simulink model "uavWaypointFollowing_HIL"  (R2021a)
settings: Solver=FixedStepDiscrete  StartTime=0.0  StopTime=10.0  RelTol=1e-3
values from neighbouring files (symbols this model uses):
  DEG2RAD = 0.0174533    [uavWaypointFollowing_HIL_Init_control.m]
  Kd_PITCH_AngleRate = 0.001    [uavWaypointFollowing_HIL_Init_control.m]
  Kd_ROLL_AngleRate = 0.001    [uavWaypointFollowing_HIL_Init_control.m]
  Kd_YAW_AngleRate = 0.00    (= 0)    [uavWaypointFollowing_HIL_Init_control.m]
  Ki_PITCH_AngleRate = 0.02    [uavWaypointFollowing_HIL_Init_control.m]
  Ki_ROLL_AngleRate = 0.02    [uavWaypointFollowing_HIL_Init_control.m]
  Ki_YAW_AngleRate = 0.001    [uavWaypointFollowing_HIL_Init_control.m]
  Kp_PITCH_ANGLE = 6.5    [uavWaypointFollowing_HIL_Init_control.m]
  Kp_PITCH_AngleRate = 0.1    [uavWaypointFollowing_HIL_Init_control.m]
  Kp_ROLL_ANGLE = 6.5    [uavWaypointFollowing_HIL_Init_control.m]
  Kp_ROLL_AngleRate = 0.1    [uavWaypointFollowing_HIL_Init_control.m]
  Kp_YAW_AngleRate = 0.3    [uavWaypointFollowing_HIL_Init_control.m]
  Kpxp = 1.0    (= 1)    [uavWaypointFollowing_HIL_Init_control.m]
  Kpyp = 1.0    (= 1)    [uavWaypointFollowing_HIL_Init_control.m]
  Kpzp = 4.0    (= 4)    [uavWaypointFollowing_HIL_Init_control.m]
  Kvxd = 0.01    [uavWaypointFollowing_HIL_Init_control.m]
  Kvxi = 0.4    [uavWaypointFollowing_HIL_Init_control.m]
  Kvxp = 2.5    [uavWaypointFollowing_HIL_Init_control.m]
  Kvyd = 0.01    [uavWaypointFollowing_HIL_Init_control.m]
  Kvyi = 0.4    [uavWaypointFollowing_HIL_Init_control.m]
  Kvyp = 2.5    [uavWaypointFollowing_HIL_Init_control.m]
  Kvzd = 0.005    [uavWaypointFollowing_HIL_Init_control.m]
  Kvzi = 0.01    [uavWaypointFollowing_HIL_Init_control.m]
  Kvzp = 0.45    [uavWaypointFollowing_HIL_Init_control.m]
  MAX_CONTROL_ANGLE_PITCH = 35    [uavWaypointFollowing_HIL_Init_control.m]
  MAX_CONTROL_ANGLE_RATE_PITCH = 220    [uavWaypointFollowing_HIL_Init_control.m]
  MAX_CONTROL_ANGLE_RATE_ROLL = 220    [uavWaypointFollowing_HIL_Init_control.m]
  MAX_CONTROL_ANGLE_RATE_Y = 200    [uavWaypointFollowing_HIL_Init_control.m]
  MAX_CONTROL_ANGLE_ROLL = 35    [uavWaypointFollowing_HIL_Init_control.m]
  MAX_CONTROL_VELOCITY_XY = 5    [uavWaypointFollowing_HIL_Init_control.m]
  MAX_CONTROL_VELOCITY_Z = 3    [uavWaypointFollowing_HIL_Init_control.m]
  Saturation_I_ah = 3.43    [uavWaypointFollowing_HIL_Init_control.m]
  Saturation_I_az = 5    [uavWaypointFollowing_HIL_Init_control.m]
  Saturation_I_RP_Max = 0.3    [uavWaypointFollowing_HIL_Init_control.m]
  Saturation_I_RP_Min = -0.3    [uavWaypointFollowing_HIL_Init_control.m]
  Saturation_I_Y_Max = 0.2    [uavWaypointFollowing_HIL_Init_control.m]
  Saturation_I_Y_Min = -0.2    [uavWaypointFollowing_HIL_Init_control.m]
  THR_HOVER = 0.609    [uavWaypointFollowing_HIL_Init_control.m]
undefined symbols (not defined in the file or in its folder): DiscIntNeverNeededParam, RGBLED_COLOR_ENUM, RGBLED_MODE_ENUM
libraries: simulink x7, pixhawk_slib_sensors_actuators x4, pixhawk_slib_uORB_RW x2
(part 2 of 2)

== matlab function uavWaypointFollowing_HIL/Control System/Subsystem/position_control/MATLAB Function ==
  data: eax input; eay input; psi input; phi output; theta output
function [phi, theta] = fcn(eax, eay, psi)
%Function description:
%  Convert the desired horizontal acceleration to the desired attitude angle
%Input:
%  eax, eaxy: desired horizontal acceleration
%  psi: yaw
%Output:
%  phi, theta: desired roll angle and desired pitch angle
g = 9.8;
phi = (-sin(psi)*eax + cos(psi)*eay)/g;
theta = (-cos(psi)*eax - sin(psi)*eay)/g;

== matlab function uavWaypointFollowing_HIL/Control System/InputConditioning1/deadzone4 ==
  data: u input; y output
function y = fcn(u)
%Function description:
%  Control the range of the remote control input from RCMin to RCMax, and
%  set a dead zone with a dead zone size of ±deadZone. The output y is
%  normalized to 0~1.You can get the RC calibration parameters in QGC.
RCMin = 1100;
RCMax = 1900;
RCMid = (RCMin + RCMax)/2;
deadZoneRate = 0.05;
deadZone = deadZoneRate*(RCMax - RCMin);
k = 1/(RCMax - RCMid - deadZone);
% saturation
if(u < RCMin)
    u = RCMin;
elseif(u > RCMax)
    u = RCMax;
end
% dead zone and normalize
 if(u > RCMid + deadZone)
    y = (u-RCMid - deadZone)*k;
 elseif(u < RCMid - deadZone)
     y = (u - RCMid + deadZone)*k;
 else
     y = 0;
 end

 end
